simulink model "sim_system_lin_retour_etat"  (Simulink 7.9)
settings: Solver=ode45  StartTime=0.0  StopTime=t_simu  RelTol=1e-3
values from neighbouring files (symbols this model uses):
  A_lin = J    [linearisation.m]
  B_lin = [B_lin_Wf B_lin_Ccharge]    [linearisation.m]
  C_lin = [0 1 0 ... (first row only)    [linearisation.m]
  D_lin = [0 0 ... (first row only)    [linearisation.m]
  K_feedback_1 = place(A_lin, B_lin(:,1), poles_goal)    [main.m]    (also in retour_etat_simple.m)
  ss_capteur_temperature = ss(A_capteur_temperature, B_capteur_temperature, C_capteur_temperature, D_capteur_temperature)    [ss_doseur_capteur.m]
  T45_0 = f_t45(Wf_0, Ng_0)    [point_equilibre.m]
  t_step = t_simu / 2    (= 50)    [main.m]    (also in retour_etat_augmente.m; retour_etat_simple.m = 12.5)
libraries: simulink x1
settings Model: Creator=maffre  LastModifiedBy=maffre

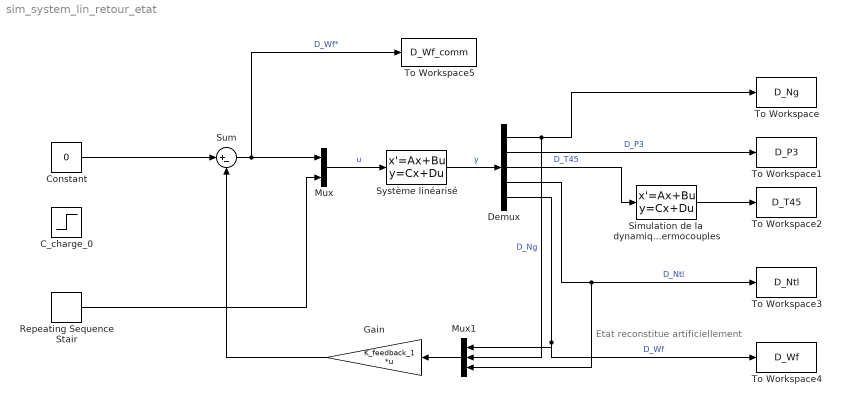
== system sim_system_lin_retour_etat ==
  note: Etat reconstitue artificiellement
  C_charge_0 : Step  Time=t_step  After=0.1  SampleTime=0
  Constant : Constant  Value=0
  Demux : Demux  Outputs=5
  Gain : Gain  Gain=K_feedback_1  Multiplication=Matrix(K*u)
  Mux : Mux  Inputs=2
  Mux1 : Mux  Inputs=3
  Repeating Sequence Stair : simulink/Sources/Repeating Sequence Stair  OutValues=[0 1 1 0].'  tsamp=10  OutMin=[]  OutMax=[]  OutDataTypeStr=double  OutputDataTypeScalingMode=double  OutDataType=fixdt(0,8)  ConRadixGroup=Best Precision: Vector-wise  OutScaling=2^-12
  Simulation de la  dynamique des  thermocouples : StateSpace  A=ss_capteur_temperature.A  B=ss_capteur_temperature.B  C=ss_capteur_temperature.C  D=ss_capteur_temperature.D  X0=T45_0
  Sum : Sum  Inputs=|+-
  Système linéarisé : StateSpace  A=A_lin  B=B_lin  C=[C_lin ; 1 0 0]  D=[D_lin ; 0 0]
  To Workspace : ToWorkspace  VariableName=D_Ng  SampleTime=-1  SaveFormat=Timeseries
  To Workspace1 : ToWorkspace  VariableName=D_P3  SampleTime=-1  SaveFormat=Timeseries
  To Workspace2 : ToWorkspace  VariableName=D_T45  SampleTime=-1  SaveFormat=Timeseries
  To Workspace3 : ToWorkspace  VariableName=D_Ntl  SampleTime=-1  SaveFormat=Timeseries
  To Workspace4 : ToWorkspace  VariableName=D_Wf  SampleTime=-1  SaveFormat=Timeseries
  To Workspace5 : ToWorkspace  VariableName=D_Wf_comm  SampleTime=-1  SaveFormat=Timeseries
  wires:
  Système linéarisé/1 -> Demux/1  "y"
  Demux/1 -> To Workspace/1, Mux1/2  "D_Ng"
  Demux/2 -> To Workspace1/1  "D_P3"
  Demux/4 -> To Workspace3/1, Mux1/3  "D_Ntl"
  Mux/1 -> Système linéarisé/1  "u"
  Simulation de la  dynamique des  thermocouples/1 -> To Workspace2/1
  Demux/3 -> Simulation de la  dynamique des  thermocouples/1  "D_T45"
  Demux/5 -> To Workspace4/1, Mux1/1  "D_Wf"
  Mux1/1 -> Gain/1
  Sum/1 -> Mux/1, To Workspace5/1  "D_Wf*"
  Gain/1 -> Sum/2
  Constant/1 -> Sum/1
  Repeating Sequence Stair/1 -> Mux/2
